simulink model "Labor_2_Aufgabe_2_c"  (R2023b)
settings: Solver=VariableStepAuto  StartTime=0.0  StopTime=10.0  RelTol=1e-3
values from neighbouring files (symbols this model uses):
  AB = 0.0226    [Laborversuch_2_skript_c.m]
  C = 0.003    [Laborversuch_2_skript_c.m]
  KR = 0.01    [Laborversuch_2_skript_c.m]
  TN = TN_array(count)    [Laborversuch_2_skript_c.m]
settings Model: Creator=danie  LastModifiedBy=danie

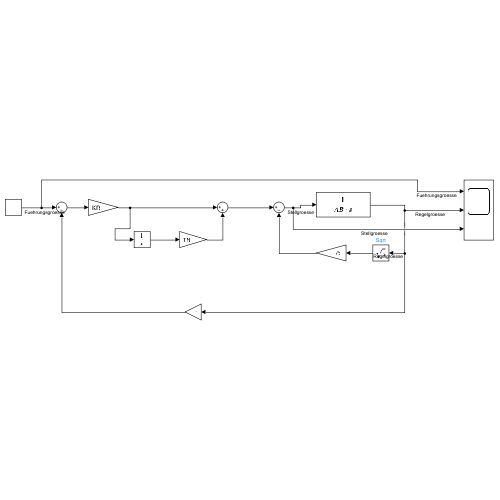
[thumbnail: Simulink's stored preview of the top-level diagram]
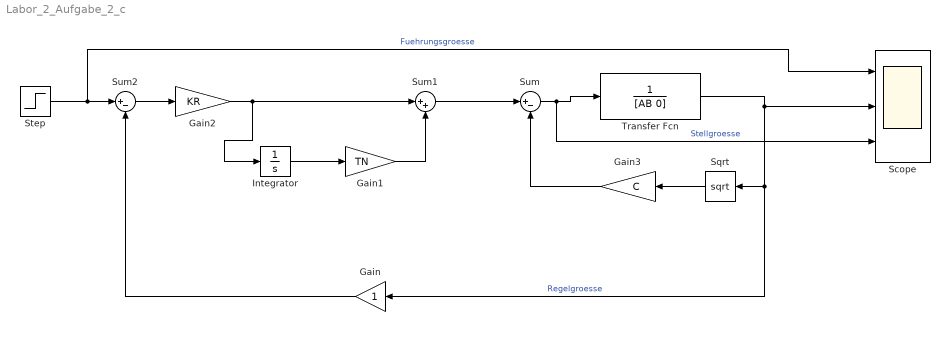
== system Labor_2_Aufgabe_2_c ==
  Gain : Gain
  Gain1 : Gain  Gain=TN
  Gain2 : Gain  Gain=KR
  Gain3 : Gain  Gain=C
  Integrator : Integrator
  Scope : Scope  NumInputPorts=3
  Sqrt : Sqrt
  Step : Step  Time=40  Before=0.1  After=0  SampleTime=0
  Sum : Sum  Inputs=|+-
  Sum1 : Sum  Inputs=|++
  Sum2 : Sum  Inputs=|+-
  Transfer Fcn : TransferFcn  Denominator=[AB 0]
  wires:
  Integrator/1 -> Gain1/1
  Step/1 -> Scope/1, Sum2/1  "Fuehrungsgroesse"
  Sum2/1 -> Gain2/1
  Gain2/1 -> Integrator/1, Sum1/1
  Gain1/1 -> Sum1/2
  Sum1/1 -> Sum/1
  Gain3/1 -> Sum/2
  Sqrt/1 -> Gain3/1
  Sum/1 -> Scope/3, Transfer Fcn/1  "Stellgroesse"
  Transfer Fcn/1 -> Scope/2, Gain/1, Sqrt/1  "Regelgroesse"
  Gain/1 -> Sum2/2
